simulink model "Spring_Mass_Damper"  (R2021b)
settings: Solver=VariableStepAuto  StartTime=0.0  StopTime=10.0  RelTol=1e-3
values from neighbouring files (symbols this model uses):
  c1 = 1    [Spring_Mass_Damper_Variables.m]
  k = 200000    [FreeVibrationResponse.m]    (also in Spring_Mass_Damper_Variables.m = 10)
  m = 500    [FreeVibrationResponse.m]    (also in Spring_Mass_Damper_Variables.m = 2)
settings Model: Creator=ammo5  LastModifiedBy=ammo5

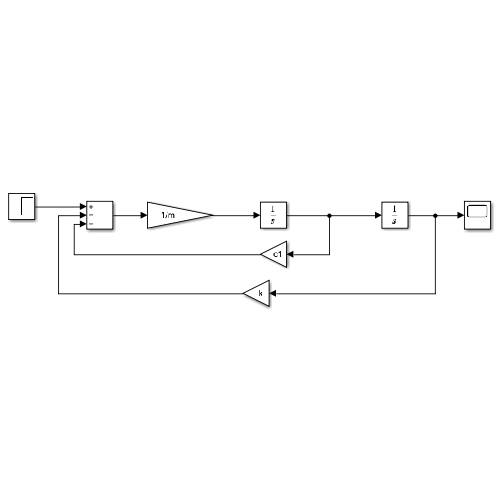
[thumbnail: Simulink's stored preview of the top-level diagram]
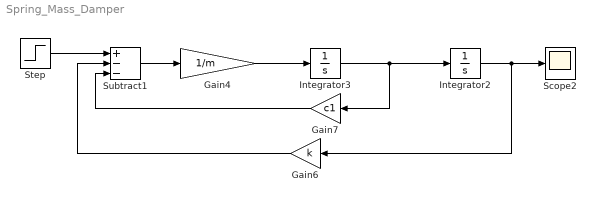
== system Spring_Mass_Damper ==
  Gain4 : Gain  Gain=1/m
  Gain6 : Gain  Gain=k
  Gain7 : Gain  Gain=c1
  Integrator2 : Integrator
  Integrator3 : Integrator
  Scope2 : Scope
  Step : Step  SampleTime=0
  Subtract1 : Sum  Inputs=+--
  wires:
  Integrator2/1 -> Scope2/1, Gain6/1
  Gain6/1 -> Subtract1/2
  Subtract1/1 -> Gain4/1
  Gain4/1 -> Integrator3/1
  Gain7/1 -> Subtract1/3
  Integrator3/1 -> Integrator2/1, Gain7/1
  Step/1 -> Subtract1/1
